simulink model "llms"  (Simulink 7.3)
settings: Solver=FixedStepDiscrete  StartTime=0.0  StopTime=10.0  RelTol=1e-3
settings Model: Creator=HP  LastModifiedBy=HP
settings SolverCC: ZeroCrossAlgorithm=Adaptive

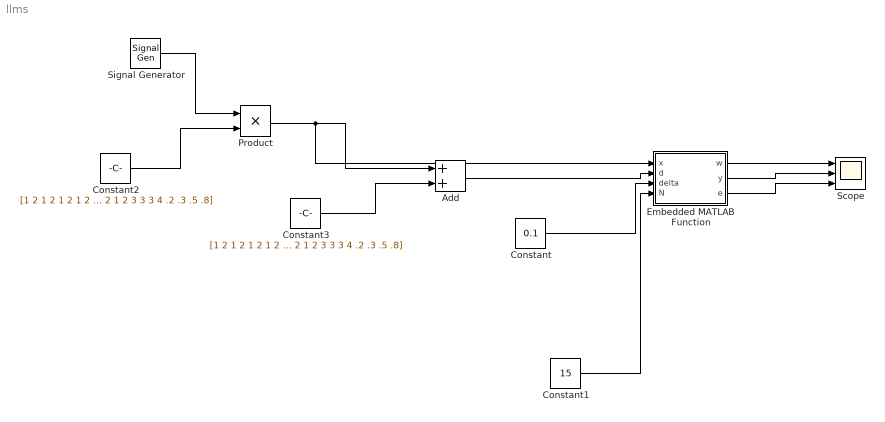
== system llms ==
  Add : Sum  OutDataType=fixdt(1, 16)  OutScaling=2^-10
  Constant : Constant  Value=0.1  OutDataType=fixdt(1, 16)  OutScaling=2^0
  Constant1 : Constant  Value=15  OutDataType=fixdt(1, 16)  OutScaling=2^0
  Constant2 : Constant  Value=[1 2 1 2 1 2 1 2 1 2 1 2 3 3 3 4 .2 .3 .5 .8]  OutDataType=fixdt(1, 16)  OutScaling=2^0
  Constant3 : Constant  Value=[1 2 1 2 1 2 1 2 1 2 1 2 3 3 3 4 .2 .3 .5 .8]  OutDataType=fixdt(1, 16)  OutScaling=2^0
  Embedded MATLAB Function : Stateflow chart
  Product : Product  OutDataType=fixdt(1, 16)  OutScaling=2^0  RndMeth=Zero
  Scope : Scope  NumInputPorts=3
      settings: YMin=-5~-5~-5  YMax=5~5~5
  Signal Generator : SignalGenerator  Frequency=50
  wires:
  Add/1 -> Embedded MATLAB Function/2(d)
  Constant3/1 -> Add/2
  Constant1/1 -> Embedded MATLAB Function/4(N)
  Constant/1 -> Embedded MATLAB Function/3(delta)
  Signal Generator/1 -> Product/1
  Constant2/1 -> Product/2
  Product/1 -> Add/1, Embedded MATLAB Function/1(x)
  Embedded MATLAB Function/1(w) -> Scope/1
  Embedded MATLAB Function/2(y) -> Scope/2
  Embedded MATLAB Function/3(e) -> Scope/3

== matlab function Embedded MATLAB Function ==
  settings: updateMethod=DISCRETE  sampleTime=1
  data: x input double size=[1 20]; d input double size=[1 20]; w output double size=[1 15]; y output double size=20; delta input double size=1; e output double size=1; N input double size=1
function [w,y,e ] = lmsa(x,d,delta,N)
%#eml
M=length(x);
N=15;
M=20;
w=zeros(1,N);
x1=zeros(1,N);
for n=N:M;
    x1=x(n:-1:n-N+1);
    y=w*x1';
    e=d(n)-y;
    w=w+delta*e*x1;
end
    N=15;
delta=0.1;
x=randn(1,20);
d=x+randn(1,20);
eml.extrinsic('lmsa')
[w,y,e ] = lmsa( x,d,delta,N)
